simulink model "Ex_06"  (R2020b)
settings: Solver=ode3  StartTime=0.0  StopTime=10  FixedStep=1  RelTol=1e-3  EnableMultiTasking=on
settings Model: Creator=Vesely  LastModifiedBy=Ludek
settings DataIOCC: LimitDataPoints=on  SaveFormat=Array  SignalLoggingSaveFormat=ModelDataLogs  ReturnWorkspaceOutputs=off
settings OptimizationCC: ExpressionDepthLimit=2147483647  LifeSpan=inf
settings DebuggingCC: UnderspecifiedInitializationDetection=Classic  MergeDetectMultiDrivingBlocksExec=none  SolverPrmCheckMsg=warning  FcnCallInpInsideContextMsg=warning  AllowSymbolicDim=off  StateNameClashWarn=warning  SFUnexpectedBacktrackingDiag=warning  SFNoUnconditionalDefaultTransitionDiag=warning  SFExecutionAtInitializationDiag=none  ArithmeticOperatorsInVariantConditions=warning
settings HardwareCC: ProdBitPerPointer=32  ProdBitPerSizeT=32  ProdBitPerPtrDiffT=32  ProdLargestAtomicFloat=None  ProdIntDivRoundTo=Undefined  ProdEndianess=Unspecified  ProdWordSize=32  ProdHWDeviceType=32-bit Generic
settings ModelReferenceCC: PropagateSignalLabelsOutOfModel=off
settings SFSimCC: SimUseLocalCustomCode=off  CustomCodeUndefinedFunction=UseInterfaceOnly
settings RTWCC: RTWUseLocalCustomCode=off
settings CodeAppCC: StateflowObjectComments=on
settings GRTTargetCC: TargetLangStandard=C89/C90 (ANSI)  CombineOutputUpdateFcns=off  GRTInterface=on
settings ConfigComp: CovMetricSettings=dw  CovSaveCumulativeToWorkspaceVar=on  CovSaveSingleToWorkspaceVar=on  CovExternalEMLEnable=off

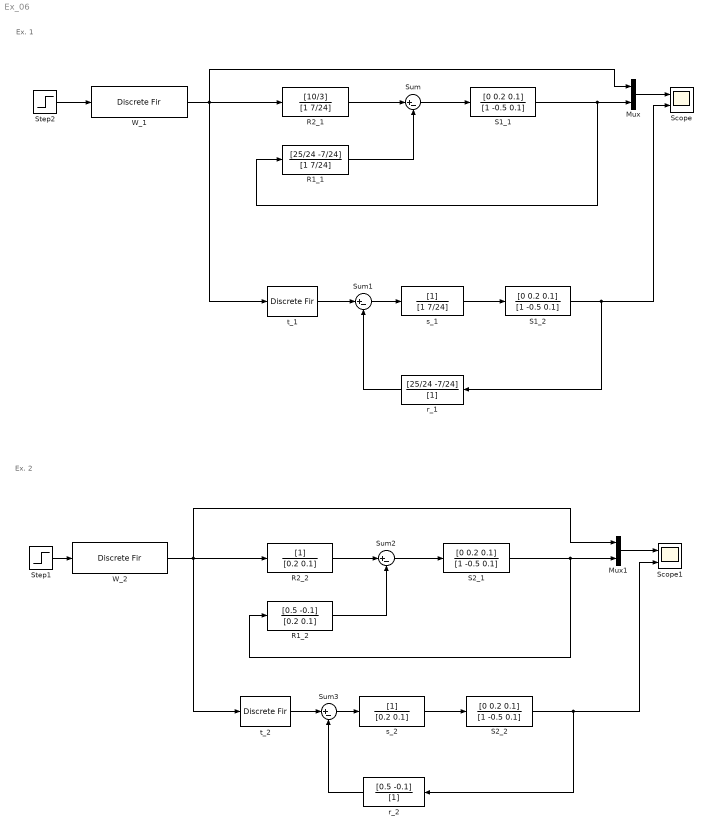
== system Ex_06 ==
  note: Ex. 2
  note: Ex. 1
  Mux : Mux  Inputs=2
  Mux1 : Mux  Inputs=2
  R1_1 : DiscreteFilter  Numerator=[25/24 -7/24]  Denominator=[1 7/24]
  R1_2 : DiscreteFilter  Numerator=[0.5 -0.1]  Denominator=[0.2 0.1]
  R2_1 : DiscreteFilter  Numerator=[10/3]  Denominator=[1 7/24]
  R2_2 : DiscreteFilter  Denominator=[0.2 0.1]
  S1_1 : DiscreteFilter  Numerator=[0 0.2 0.1]  Denominator=[1 -0.5 0.1]
  S1_2 : DiscreteFilter  Numerator=[0 0.2 0.1]  Denominator=[1 -0.5 0.1]
  S2_1 : DiscreteFilter  Numerator=[0 0.2 0.1]  Denominator=[1 -0.5 0.1]
  S2_2 : DiscreteFilter  Numerator=[0 0.2 0.1]  Denominator=[1 -0.5 0.1]
  Scope : Scope  NumInputPorts=2
  Scope1 : Scope  NumInputPorts=2
  Step1 : Step  Before=1  After=0
  Step2 : Step  Before=1  After=0
  Sum{,1..3} (4 alike) : Sum  Inputs=|+-
  W_1 : DiscreteFir  Coefficients=[1 1 1 1 1 ]  AccumDataTypeStr=Inherit: Same as product output
  W_2 : DiscreteFir  Coefficients=[1 1 1 1 1 ]  AccumDataTypeStr=Inherit: Same as product output
  r_1 : DiscreteFilter  Numerator=[25/24 -7/24]  Denominator=[1]
  r_2 : DiscreteFilter  Numerator=[0.5 -0.1]  Denominator=[1]
  s_1 : DiscreteFilter  Denominator=[1 7/24]
  s_2 : DiscreteFilter  Denominator=[0.2 0.1]
  t_1 : DiscreteFir  Coefficients=[10/3]  AccumDataTypeStr=Inherit: Same as product output
  t_2 : DiscreteFir  Coefficients=[1]  AccumDataTypeStr=Inherit: Same as product output
  wires:
  Step2/1 -> W_1/1
  R2_1/1 -> Sum/1
  Sum/1 -> S1_1/1
  R1_1/1 -> Sum/2
  S1_1/1 -> R1_1/1, Mux/2
  W_1/1 -> R2_1/1, Mux/1, t_1/1
  t_1/1 -> Sum1/1
  Sum1/1 -> s_1/1
  S1_2/1 -> Scope/2, r_1/1
  s_1/1 -> S1_2/1
  r_1/1 -> Sum1/2
  Step1/1 -> W_2/1
  R2_2/1 -> Sum2/1
  Sum2/1 -> S2_1/1
  R1_2/1 -> Sum2/2
  S2_1/1 -> R1_2/1, Mux1/2
  Mux/1 -> Scope/1
  Mux1/1 -> Scope1/1
  S2_2/1 -> r_2/1, Scope1/2
  W_2/1 -> R2_2/1, Mux1/1, t_2/1
  Sum3/1 -> s_2/1
  s_2/1 -> S2_2/1
  t_2/1 -> Sum3/1
  r_2/1 -> Sum3/2
